simulink model "a1"  (R2015a)
settings: Solver=ode45  StartTime=0.0  StopTime=10.0  RelTol=1e-3
settings Model: Creator=leon  LastModifiedBy=leon

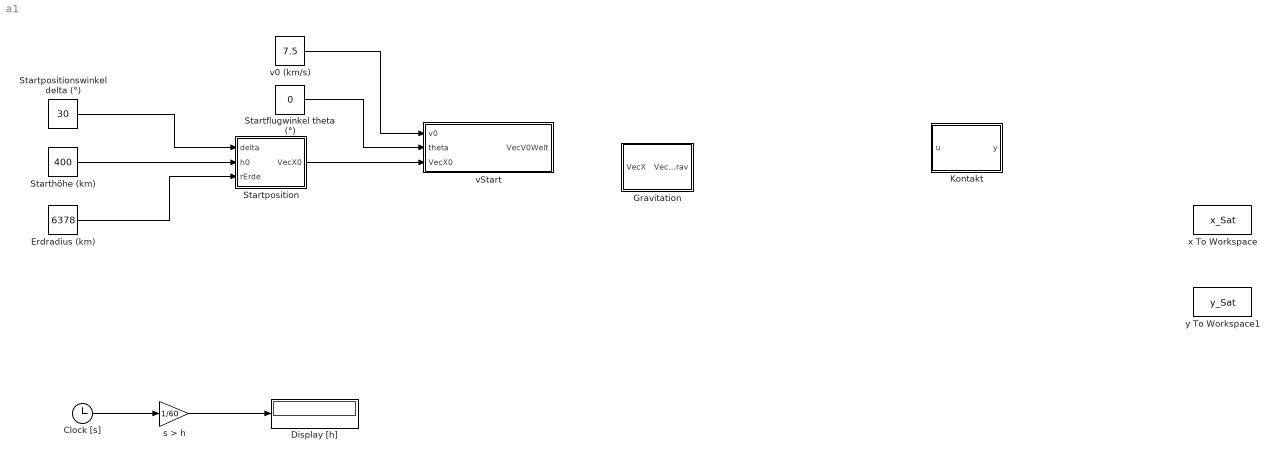
== system a1 ==
  Clock [s] : Clock
  Display [h] : Display
  "Erdradius (km) " : Constant  Value=6378
  Gravitation : MATLAB Function  TreatAsAtomicUnit=on
  Kontakt : MATLAB Function  TreatAsAtomicUnit=on
  Startflugwinkel theta (°) : Constant  Value=0
  Starthöhe (km) : Constant  Value=400
  Startposition : MATLAB Function  TreatAsAtomicUnit=on
  "Startpositionswinkel delta (°) " : Constant  Value=30
  s > h : Gain  Gain=1/60
  v0 (km/s) : Constant  Value=7.5
  vStart : MATLAB Function  TreatAsAtomicUnit=on
  x To Workspace : ToWorkspace  VariableName=x_Sat  SampleTime=-1
  y To Workspace1 : ToWorkspace  VariableName=y_Sat  SampleTime=-1
  wires:
  Startposition/1(VecX0) -> vStart/3(VecX0)
  "Startpositionswinkel delta (°) "/1 -> Startposition/1(delta)
  Starthöhe (km)/1 -> Startposition/2(h0)
  "Erdradius (km) "/1 -> Startposition/3(rErde)
  Startflugwinkel theta (°)/1 -> vStart/2(theta)
  v0 (km/s)/1 -> vStart/1(v0)
  Clock [s]/1 -> s > h/1
  s > h/1 -> Display [h]/1

== matlab function a1/vStart ==
  data: v0 input; VecV0Welt output; theta input; VecX0 input
function VecV0Welt = fcn(v0, theta, VecX0)
%#codegen
VecV0Welt = [0,1,2];

== matlab function a1/Startposition ==
  data: delta input; VecX0 output; h0 input; rErde input
%Geben Sie eine Embedded-Matlab-(EM)-Funktion „Startposition“ an,
%die aus den Parametern (°), der Starthöhe h 0 (km) sowie der Konstante „Erdradius“
%die Startposition ⃗ berechnet ( Anfangswert für die Position).

function VecX0 = fcn(delta, h0, rErde)
VecX0 = [0, 1,2];

%#codegen

== matlab function a1/Gravitation ==
  data: VecX input; VecGrav output
function VecGrav = fcn(VecX)
%#codegen

VecGrav = [0,1,2];

== matlab function a1/Kontakt ==
  data: u input; y output
function y = fcn(u)
%#codegen

y = u;
